simulink model "c12_ConsensusMultiDelaysModel"  (R2020b)
settings: Solver=VariableStepAuto  StartTime=0.0  StopTime=t_end  MaxStep=0.01  MinStep=0.001  RelTol=1e-3
values from neighbouring files (symbols this model uses):
  L1 = Hbar1'*W*Hbar1    [c12_MultipleDelaysLMI.m]
  L2 = Hbar2'*W*Hbar2    [c12_MultipleDelaysLMI.m]
  L3 = Hbar3'*W*Hbar3    [c12_MultipleDelaysLMI.m]
  x0 = 5    [c12_delayAdaptive.m]    (also in c14_bipartite_MWconsensus_animation.m = [x0;r/norm(r)]; c15_closed_model.m = 5*rand(15,1); c15_open_model.m = 5*rand(15,1))
undefined symbols (not defined in the file or in its folder): tau1, tau2, tau3
settings Model: Creator=HoangMinh  LastModifiedBy=trinh

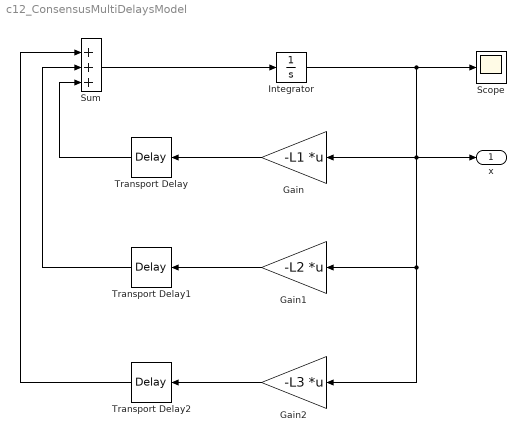
== system c12_ConsensusMultiDelaysModel ==
  Gain : Gain  Gain=-L1  Multiplication=Matrix(K*u) (u vector)
  Gain1 : Gain  Gain=-L2  Multiplication=Matrix(K*u) (u vector)
  Gain2 : Gain  Gain=-L3  Multiplication=Matrix(K*u) (u vector)
  Integrator : Integrator  InitialCondition=x0
  Scope : Scope
  Sum : Sum  Inputs=|+++
  Transport Delay : TransportDelay  DelayTime=tau1
  Transport Delay1 : TransportDelay  DelayTime=tau2
  Transport Delay2 : TransportDelay  DelayTime=tau3
  x : Outport  SignalName=x
  wires:
  Gain/1 -> Transport Delay/1
  Gain2/1 -> Transport Delay2/1
  Transport Delay2/1 -> Sum/1
  Gain1/1 -> Transport Delay1/1
  Transport Delay1/1 -> Sum/2
  Integrator/1 -> Scope/1, x/1, Gain2/1, Gain1/1, Gain/1
  Sum/1 -> Integrator/1
  Transport Delay/1 -> Sum/3
